simulink model "hexapod"  (R2022a)
settings: Solver=ode2  StartTime=0.0  StopTime=10.0  FixedStep=1e-4  RelTol=1e-3  AbsTol=1e-3  EnableMultiTasking=on
values from neighbouring files (symbols this model uses):
  N = 2    [gen_singleGait.m]
  s = t/T    [gait_mv_backward.m]    (also in gait_mv_forward.m; gait_mv_left.m; gait_mv_right.m; gait_rot_clockwise.m)
undefined symbols (not defined in the file or in its folder): X, Y, Z
libraries: sm_lib x90, nesl_utility x19, Contact_Forces_Lib x6, simulink x1
(part 4 of 4)

== matlab function hexapod/Leg6/MATLAB Function ==
  data: i input; ang1 output; x0 input; y0 input; z0 input; ang2 output; ang3 output; theta1 input; theta2 input; theta3 input; l1 input; l2 input; l3 input; xx1 input; yy1 input; yy2 input
function [ang1,ang2,ang3] = fcn(i,x0,y0,z0,theta1,theta2,theta3,l1,l2,l3,xx1,yy1,yy2)
p0=[x0;y0;z0];
p00=[p0;1];
j3bias=10.91;
% %
% PX=worldCo2jointCo(i,p0);
% ang=jointCo2jointAng(PX);
% ang
function TR=TROTZ(theta)
    r=theta/180*pi;
    TR=[cos(r),-sin(r),0,0;
        sin(r),cos(r),0,0;
        0,      0,    1,0;
        0,      0,    0,1];
end
function TL=TRANSL(x,y,z)
    TL=[1,0,0,x;
        0,1,0,y;
        0,0,1,z;
        0,0,0,1];
end

%%  p0->px
switch i
    case 1
        Tx_0=TROTZ(theta1)*TRANSL(-xx1,yy1,0);
    case 2
        Tx_0=TROTZ(-theta2)*TRANSL(0,-yy2,0);
    case 3
        Tx_0=TROTZ(theta3)*TRANSL(xx1,yy1,0);
    case 4
        Tx_0=TROTZ(-theta1)*TRANSL(-xx1,-yy1,0);
    case 5
        Tx_0=TROTZ(theta2)*TRANSL(0,yy2,0);
    case 6
        Tx_0=TROTZ(-theta3)*TRANSL(xx1,-yy1,0);
    otherwise
        Tx_0=zeros(4);
        disp("jijiji");
end
% Tx_0

pxx=Tx_0*p00;
px=pxx(1:3,1);
% disp(p00)
% disp(pxx)
%% px->ang
x=px(1);
y=px(2);
z=px(3);
A=sqrt(x*x+y*y)-l1;
B=-z;
if(A>0)
        assert((A*A+(z-l2)*(z-l2))>l3*l3,"not in the workspace!");
        assert((A*A+z*z)<(l2+l3)*(l2+l3),"not in the workspace!");
else
    assert((A*A+z*z)>(l3-l2)*(l3-l2),"not in the workspace!");
    assert((A*A+(z+l2)*(z+l2))<l3*l3,"not in the workspace!");
end

   

    %% 
    %   r1
    r1=atan2(y,x)*(180/pi);
        assert(r1>-60,"r1<-60, dangerous!");
        assert(r1<60,"r1>60, dangerous!");

    if((A*A+z*z)>(l2*l2+l3*l3))
%         disp("高机位捏");
            %r3
            ccos=acos((l2*l2+l3*l3-A*A-B*B)/(2*l2*l3))*(180/pi);
            if(ccos>90)
                ccos=180-ccos;
            end
            r3=180-ccos-j3bias;
                assert(r3>90-j3bias,"r3<79.09, dangerous! (might be solution of low position)");
                assert(r3<(180-j3bias),"r3>169.09, dangerous!");
            %r2
            delta=atan((l3*sin(ccos/180*pi))/(l2+(l3*cos(ccos/180*pi))));
            ttan=atan(B/A);
            r2=-90-(ttan-delta)/pi*180;
                assert(r2<0,"r2>0, dangerous!")
                assert(r2>-180,"r2<-180, dangerous!")

    else
%         disp("低机位捏");
            %   r2 
            ccos=acos((A*A+B*B+l2*l2-l3*l3)/(2*sqrt(A*A+B*B)*l2))*(180/pi);
            r2=ccos-(atan2(B,A)*(180/pi))-90;
                assert(r2>=-180,"r2<=-180, dangerous!");
                assert(r2<0,"r2>0, dangerous!");
            %   r3
            ccos2=acos((-A*A-B*B+l2*l2+l3*l3)/(2*l2*l3))*(180/pi);
                if ccos2>=90
                    ccos2=180-ccos2;
                end
            r3=ccos2-j3bias;
                assert(r3>0,"r3<0, dangerous!");
                assert(r3<(90-j3bias),"r3>79.09, dangerous!(might be solution of high position)");
                
    end

%%
ang1=r1/180*pi;
ang2=r2/180*pi;
ang3=r3/180*pi;
end

== matlab function hexapod/gait generator/前进步态/前进步态 ==
  data: x1 input; ox1 output; x2 input; z1 input; z2 input; ox2 output; ox3 output; ox4 output; ox5 output; ox6 output; oy1 output; oy2 output; oy3 output; oy4 output; oy5 output; oy6 output; oz1 output; oz2 output; oz3 output; oz4 output; oz5 output; oz6 output; xxx1 input; yyy1 input; yyy2 input; zzz1 input
function [ox1,ox2,ox3,ox4,ox5,ox6,oy1,oy2,oy3,oy4,oy5,oy6,oz1,oz2,oz3,oz4,oz5,oz6] = fcn(x1,x2,z1,z2,xxx1,yyy1,yyy2,zzz1)
% baseBias={[xxx1;-yyy1;zzz1],   [0;yyy2;zzz1],   [-xxx1;-yyy1;zzz1],...
%            [xxx1;yyy1;zzz1],    [0;-yyy2;zzz1],  [-xxx1;yyy1;zzz1]};
ox1= xxx1+x1;
ox2=      x1;
ox3=-xxx1+x1;
ox4= xxx1+x2;
ox5=      x2;
ox6=-xxx1+x2;

oy1=-yyy1;
oy2=yyy2;
oy3=-yyy1;
oy4=yyy1;
oy5=-yyy2;
oy6=yyy1;

oz1=zzz1+z1;
oz2=zzz1+z1;
oz3=zzz1+z1;
oz4=zzz1+z2;
oz5=zzz1+z2;
oz6=zzz1+z2;

== matlab function hexapod/gait generator/右移步态/步态函数 ==
  data: x1 input; ox1 output; x2 input; z1 input; z2 input; ox2 output; ox3 output; ox4 output; ox5 output; ox6 output; oy1 output; oy2 output; oy3 output; oy4 output; oy5 output; oy6 output; oz1 output; oz2 output; oz3 output; oz4 output; oz5 output; oz6 output; xxx1 input; yyy1 input; yyy2 input; zzz1 input
function [ox1,ox2,ox3,ox4,ox5,ox6,oy1,oy2,oy3,oy4,oy5,oy6,oz1,oz2,oz3,oz4,oz5,oz6] = fcn(x1,x2,z1,z2,xxx1,yyy1,yyy2,zzz1)
% baseBias={[xxx1;-yyy1;zzz1],   [0;yyy2;zzz1],   [-xxx1;-yyy1;zzz1],...
%            [xxx1;yyy1;zzz1],    [0;-yyy2;zzz1],  [-xxx1;yyy1;zzz1]};
ox1= xxx1;
ox2=0;
ox3=-xxx1;
ox4= xxx1;
ox5=0;
ox6=-xxx1;

oy1=-yyy1-x1;
oy2=yyy2-x1;
oy3=-yyy1-x1;
oy4=yyy1-x2;
oy5=-yyy2-x2;
oy6=yyy1-x2;

oz1=zzz1+z1;
oz2=zzz1+z1;
oz3=zzz1+z1;
oz4=zzz1+z2;
oz5=zzz1+z2;
oz6=zzz1+z2;

== matlab function hexapod/gait generator/后退步态/步态函数 ==
  data: x1 input; ox1 output; x2 input; z1 input; z2 input; ox2 output; ox3 output; ox4 output; ox5 output; ox6 output; oy1 output; oy2 output; oy3 output; oy4 output; oy5 output; oy6 output; oz1 output; oz2 output; oz3 output; oz4 output; oz5 output; oz6 output; xxx1 input; yyy1 input; yyy2 input; zzz1 input
function [ox1,ox2,ox3,ox4,ox5,ox6,oy1,oy2,oy3,oy4,oy5,oy6,oz1,oz2,oz3,oz4,oz5,oz6] = fcn(x1,x2,z1,z2,xxx1,yyy1,yyy2,zzz1)
% baseBias={[xxx1;-yyy1;zzz1],   [0;yyy2;zzz1],   [-xxx1;-yyy1;zzz1],...
%            [xxx1;yyy1;zzz1],    [0;-yyy2;zzz1],  [-xxx1;yyy1;zzz1]};
ox1= xxx1-x1;
ox2=     -x1;
ox3=-xxx1-x1;
ox4= xxx1-x2;
ox5=     -x2;
ox6=-xxx1-x2;

oy1=-yyy1;
oy2=yyy2;
oy3=-yyy1;
oy4=yyy1;
oy5=-yyy2;
oy6=yyy1;

oz1=zzz1+z1;
oz2=zzz1+z1;
oz3=zzz1+z1;
oz4=zzz1+z2;
oz5=zzz1+z2;
oz6=zzz1+z2;

== matlab function hexapod/gait generator/左移步态/步态函数 ==
  data: x1 input; ox1 output; x2 input; z1 input; z2 input; ox2 output; ox3 output; ox4 output; ox5 output; ox6 output; oy1 output; oy2 output; oy3 output; oy4 output; oy5 output; oy6 output; oz1 output; oz2 output; oz3 output; oz4 output; oz5 output; oz6 output; xxx1 input; yyy1 input; yyy2 input; zzz1 input
function [ox1,ox2,ox3,ox4,ox5,ox6,oy1,oy2,oy3,oy4,oy5,oy6,oz1,oz2,oz3,oz4,oz5,oz6] = fcn(x1,x2,z1,z2,xxx1,yyy1,yyy2,zzz1)
% baseBias={[xxx1;-yyy1;zzz1],   [0;yyy2;zzz1],   [-xxx1;-yyy1;zzz1],...
%            [xxx1;yyy1;zzz1],    [0;-yyy2;zzz1],  [-xxx1;yyy1;zzz1]};
ox1= xxx1;
ox2=0;
ox3=-xxx1;
ox4= xxx1;
ox5=0;
ox6=-xxx1;

oy1=-yyy1+x1;
oy2=yyy2+x1;
oy3=-yyy1+x1;
oy4=yyy1+x2;
oy5=-yyy2+x2;
oy6=yyy1+x2;

oz1=zzz1+z1;
oz2=zzz1+z1;
oz3=zzz1+z1;
oz4=zzz1+z2;
oz5=zzz1+z2;
oz6=zzz1+z2;

== matlab function hexapod/gait generator/足尖轨迹生成/x ==
  data: t input; x output; L input
function x = fcn(t,L)
%   t值域为0-1
if t<0.5
    x=L*(-16*power(t,3)+12*power(t,2)-t-1/4);
else
    x=-L*t+0.75*L;
end

== matlab function hexapod/gait generator/足尖轨迹生成/z ==
  data: t input; z output; H input
function z = fcn(t,H)
%   t值域为0-1
if t<0.5
    if t<0.25
        z=H*(-128*power(t,3)+48*power(t,2));
    else
        z=H*(-128*power((0.5-t),3)+48*power((0.5-t),2));
    end
else
    z=0;
end

== matlab function hexapod/gait generator/逆时针旋转步态/步态函数 ==
  data: x1 input; ox1 output; x2 input; z1 input; z2 input; ox2 output; ox3 output; ox4 output; ox5 output; ox6 output; oy1 output; oy2 output; oy3 output; oy4 output; oy5 output; oy6 output; oz1 output; oz2 output; oz3 output; oz4 output; oz5 output; oz6 output; xxx1 input; yyy1 input; yyy2 input; zzz1 input; L0 input; theta1 input; theta2 input; theta3 input; Ang input
function [ox1,ox2,ox3,ox4,ox5,ox6,oy1,oy2,oy3,oy4,oy5,oy6,oz1,oz2,oz3,oz4,oz5,oz6] = fcn(x1,x2,z1,z2,xxx1,yyy1,yyy2,zzz1,L0,theta1,theta2,theta3,Ang)
% baseBias={[xxx1;-yyy1;zzz1],   [0;yyy2;zzz1],   [-xxx1;-yyy1;zzz1],...
%            [xxx1;yyy1;zzz1],    [0;-yyy2;zzz1],  [-xxx1;yyy1;zzz1]};
% theta=[theta1,-theta2,theta3,-theta1,theta2,-theta3]

LL1=sqrt(xxx1*xxx1+yyy1*yyy1);
LL2=yyy2;       %sqrt(0*0+yyy2*yyy2)
L1=sqrt(2*LL1*LL1*(1-cosd(Ang)));     %4条腿的移动距离
L2=sqrt(2*LL2*LL2*(1-cosd(Ang)));     %中间2条腿的移动距离

x1_1=-x1*(L0/L1);
x2_1=-x2*(L0/L1);
z1_1=z1;
z2_1=z2;

x1_2=-x1*(L0/L2);
x2_2=-x2*(L0/L2);
z1_2=z1;
z2_2=z2;

ox1=xxx1+x1_1*sind(theta1);
oy1=-yyy1+x1_1*cosd(theta1);
oz1=zzz1+z1_1;

ox2=0+x1_2*sind(-theta2);
oy2=yyy2+x1_2*cosd(-theta2);
oz2=zzz1+z1_2;

ox3=-xxx1+x1_1*sind(theta3);
oy3=-yyy1+x1_1*cosd(theta3);
oz3=zzz1+z1_1;

ox4=xxx1+x2_1*sind(-theta1);
oy4=yyy1+x2_1*cosd(-theta1);
oz4=zzz1+z2_1;

ox5=0+x2_2*sind(theta2);
oy5=-yyy2+x2_2*cosd(theta2);
oz5=zzz1+z2_2;

ox6=-xxx1+x2_1*sind(-theta3);
oy6=yyy1+x2_1*cosd(-theta3);
oz6=zzz1+z2_1;

== matlab function hexapod/gait generator/顺时针旋转步态/步态函数 ==
  data: x1 input; ox1 output; x2 input; z1 input; z2 input; ox2 output; ox3 output; ox4 output; ox5 output; ox6 output; oy1 output; oy2 output; oy3 output; oy4 output; oy5 output; oy6 output; oz1 output; oz2 output; oz3 output; oz4 output; oz5 output; oz6 output; xxx1 input; yyy1 input; yyy2 input; zzz1 input; L0 input; theta1 input; theta2 input; theta3 input; Ang input
function [ox1,ox2,ox3,ox4,ox5,ox6,oy1,oy2,oy3,oy4,oy5,oy6,oz1,oz2,oz3,oz4,oz5,oz6] = fcn(x1,x2,z1,z2,xxx1,yyy1,yyy2,zzz1,L0,theta1,theta2,theta3,Ang)
% baseBias={[xxx1;-yyy1;zzz1],   [0;yyy2;zzz1],   [-xxx1;-yyy1;zzz1],...
%            [xxx1;yyy1;zzz1],    [0;-yyy2;zzz1],  [-xxx1;yyy1;zzz1]};
% theta=[theta1,-theta2,theta3,-theta1,theta2,-theta3]

LL1=sqrt(xxx1*xxx1+yyy1*yyy1);
LL2=yyy2;       %sqrt(0*0+yyy2*yyy2)
L1=sqrt(2*LL1*LL1*(1-cosd(Ang)));     %4条腿的移动距离
L2=sqrt(2*LL2*LL2*(1-cosd(Ang)));     %中间2条腿的移动距离

x1_1=x1*(L0/L1);
x2_1=x2*(L0/L1);
z1_1=z1;
z2_1=z2;

x1_2=x1*(L0/L2);
x2_2=x2*(L0/L2);
z1_2=z1;
z2_2=z2;

ox1=xxx1+x1_1*sind(theta1);
oy1=-yyy1+x1_1*cosd(theta1);
oz1=zzz1+z1_1;

ox2=0+x1_2*sind(-theta2);
oy2=yyy2+x1_2*cosd(-theta2);
oz2=zzz1+z1_2;

ox3=-xxx1+x1_1*sind(theta3);
oy3=-yyy1+x1_1*cosd(theta3);
oz3=zzz1+z1_1;

ox4=xxx1+x2_1*sind(-theta1);
oy4=yyy1+x2_1*cosd(-theta1);
oz4=zzz1+z2_1;

ox5=0+x2_2*sind(theta2);
oy5=-yyy2+x2_2*cosd(theta2);
oz5=zzz1+z2_2;

ox6=-xxx1+x2_1*sind(-theta3);
oy6=yyy1+x2_1*cosd(-theta3);
oz6=zzz1+z2_1;

== matlab function hexapod/Leg1/w-leg1/MATLAB Function ==
  data: i input; ang1 output; x0 input; y0 input; z0 input; ang2 output; ang3 output; theta1 input; theta2 input; theta3 input; l1 input; l2 input; l3 input; xx1 input; yy1 input; yy2 input
function [ang1,ang2,ang3] = fcn(i,x0,y0,z0,theta1,theta2,theta3,l1,l2,l3,xx1,yy1,yy2)
p0=[x0;y0;z0];
p00=[p0;1];
j3bias=10.91;
% %
% PX=worldCo2jointCo(i,p0);
% ang=jointCo2jointAng(PX);
% ang
function TR=TROTZ(theta)
    r=theta/180*pi;
    TR=[cos(r),-sin(r),0,0;
        sin(r),cos(r),0,0;
        0,      0,    1,0;
        0,      0,    0,1];
end
function TL=TRANSL(x,y,z)
    TL=[1,0,0,x;
        0,1,0,y;
        0,0,1,z;
        0,0,0,1];
end

%%  p0->px
switch i
    case 1
        Tx_0=TROTZ(theta1)*TRANSL(-xx1,yy1,0);
    case 2
        Tx_0=TROTZ(-theta2)*TRANSL(0,-yy2,0);
    case 3
        Tx_0=TROTZ(theta3)*TRANSL(xx1,yy1,0);
    case 4
        Tx_0=TROTZ(-theta1)*TRANSL(-xx1,-yy1,0);
    case 5
        Tx_0=TROTZ(theta2)*TRANSL(0,yy2,0);
    case 6
        Tx_0=TROTZ(-theta3)*TRANSL(xx1,-yy1,0);
    otherwise
        Tx_0=zeros(4);
        disp("jijiji");
end
% Tx_0

pxx=Tx_0*p00;
px=pxx(1:3,1);
% disp(p00)
% disp(pxx)
%% px->ang
x=px(1);
y=px(2);
z=px(3);
A=sqrt(x*x+y*y)-l1;
B=-z;
if(A>0)
        assert((A*A+(z-l2)*(z-l2))>l3*l3,"not in the workspace!");
        assert((A*A+z*z)<(l2+l3)*(l2+l3),"not in the workspace!");
else
    assert((A*A+z*z)>(l3-l2)*(l3-l2),"not in the workspace!");
    assert((A*A+(z+l2)*(z+l2))<l3*l3,"not in the workspace!");
end

   

    %% 
    %   r1
    r1=atan2(y,x)*(180/pi);
        assert(r1>-60,"r1<-60, dangerous!");
        assert(r1<60,"r1>60, dangerous!");

    if((A*A+z*z)>(l2*l2+l3*l3))
%         disp("高机位捏");
            %r3
            ccos=acos((l2*l2+l3*l3-A*A-B*B)/(2*l2*l3))*(180/pi);
            if(ccos>90)
                ccos=180-ccos;
            end
            r3=180-ccos-j3bias;
                assert(r3>90-j3bias,"r3<79.09, dangerous! (might be solution of low position)");
                assert(r3<(180-j3bias),"r3>169.09, dangerous!");
            %r2
            delta=atan((l3*sin(ccos/180*pi))/(l2+(l3*cos(ccos/180*pi))));
            ttan=atan(B/A);
            r2=-90-(ttan-delta)/pi*180;
                assert(r2<0,"r2>0, dangerous!")
                assert(r2>-180,"r2<-180, dangerous!")

    else
%         disp("低机位捏");
            %   r2 
            ccos=acos((A*A+B*B+l2*l2-l3*l3)/(2*sqrt(A*A+B*B)*l2))*(180/pi);
            r2=ccos-(atan2(B,A)*(180/pi))-90;
                assert(r2>=-180,"r2<=-180, dangerous!");
                assert(r2<0,"r2>0, dangerous!");
            %   r3
            ccos2=acos((-A*A-B*B+l2*l2+l3*l3)/(2*l2*l3))*(180/pi);
                if ccos2>=90
                    ccos2=180-ccos2;
                end
            r3=ccos2-j3bias;
                assert(r3>0,"r3<0, dangerous!");
                assert(r3<(90-j3bias),"r3>79.09, dangerous!(might be solution of high position)");
                
    end

%%
ang1=r1/180*pi;
ang2=r2/180*pi;
ang3=r3/180*pi;
end

== matlab function hexapod/Leg2/w-leg1/MATLAB Function ==
  data: i input; ang1 output; x0 input; y0 input; z0 input; ang2 output; ang3 output; theta1 input; theta2 input; theta3 input; l1 input; l2 input; l3 input; xx1 input; yy1 input; yy2 input
function [ang1,ang2,ang3] = fcn(i,x0,y0,z0,theta1,theta2,theta3,l1,l2,l3,xx1,yy1,yy2)
p0=[x0;y0;z0];
p00=[p0;1];
j3bias=10.91;
% %
% PX=worldCo2jointCo(i,p0);
% ang=jointCo2jointAng(PX);
% ang
function TR=TROTZ(theta)
    r=theta/180*pi;
    TR=[cos(r),-sin(r),0,0;
        sin(r),cos(r),0,0;
        0,      0,    1,0;
        0,      0,    0,1];
end
function TL=TRANSL(x,y,z)
    TL=[1,0,0,x;
        0,1,0,y;
        0,0,1,z;
        0,0,0,1];
end

%%  p0->px
switch i
    case 1
        Tx_0=TROTZ(theta1)*TRANSL(-xx1,yy1,0);
    case 2
        Tx_0=TROTZ(-theta2)*TRANSL(0,-yy2,0);
    case 3
        Tx_0=TROTZ(theta3)*TRANSL(xx1,yy1,0);
    case 4
        Tx_0=TROTZ(-theta1)*TRANSL(-xx1,-yy1,0);
    case 5
        Tx_0=TROTZ(theta2)*TRANSL(0,yy2,0);
    case 6
        Tx_0=TROTZ(-theta3)*TRANSL(xx1,-yy1,0);
    otherwise
        Tx_0=zeros(4);
        disp("jijiji");
end
% Tx_0

pxx=Tx_0*p00;
px=pxx(1:3,1);
% disp(p00)
% disp(pxx)
%% px->ang
x=px(1);
y=px(2);
z=px(3);
A=sqrt(x*x+y*y)-l1;
B=-z;
if(A>0)
        assert((A*A+(z-l2)*(z-l2))>l3*l3,"not in the workspace!");
        assert((A*A+z*z)<(l2+l3)*(l2+l3),"not in the workspace!");
else
    assert((A*A+z*z)>(l3-l2)*(l3-l2),"not in the workspace!");
    assert((A*A+(z+l2)*(z+l2))<l3*l3,"not in the workspace!");
end

   

    %% 
    %   r1
    r1=atan2(y,x)*(180/pi);
        assert(r1>-60,"r1<-60, dangerous!");
        assert(r1<60,"r1>60, dangerous!");

    if((A*A+z*z)>(l2*l2+l3*l3))
%         disp("高机位捏");
            %r3
            ccos=acos((l2*l2+l3*l3-A*A-B*B)/(2*l2*l3))*(180/pi);
            if(ccos>90)
                ccos=180-ccos;
            end
            r3=180-ccos-j3bias;
                assert(r3>90-j3bias,"r3<79.09, dangerous! (might be solution of low position)");
                assert(r3<(180-j3bias),"r3>169.09, dangerous!");
            %r2
            delta=atan((l3*sin(ccos/180*pi))/(l2+(l3*cos(ccos/180*pi))));
            ttan=atan(B/A);
            r2=-90-(ttan-delta)/pi*180;
                assert(r2<0,"r2>0, dangerous!")
                assert(r2>-180,"r2<-180, dangerous!")

    else
%         disp("低机位捏");
            %   r2 
            ccos=acos((A*A+B*B+l2*l2-l3*l3)/(2*sqrt(A*A+B*B)*l2))*(180/pi);
            r2=ccos-(atan2(B,A)*(180/pi))-90;
                assert(r2>=-180,"r2<=-180, dangerous!");
                assert(r2<0,"r2>0, dangerous!");
            %   r3
            ccos2=acos((-A*A-B*B+l2*l2+l3*l3)/(2*l2*l3))*(180/pi);
                if ccos2>=90
                    ccos2=180-ccos2;
                end
            r3=ccos2-j3bias;
                assert(r3>0,"r3<0, dangerous!");
                assert(r3<(90-j3bias),"r3>79.09, dangerous!(might be solution of high position)");
                
    end

%%
ang1=r1/180*pi;
ang2=r2/180*pi;
ang3=r3/180*pi;
end

== matlab function hexapod/Leg3/w-leg1/MATLAB Function ==
  data: i input; ang1 output; x0 input; y0 input; z0 input; ang2 output; ang3 output; theta1 input; theta2 input; theta3 input; l1 input; l2 input; l3 input; xx1 input; yy1 input; yy2 input
function [ang1,ang2,ang3] = fcn(i,x0,y0,z0,theta1,theta2,theta3,l1,l2,l3,xx1,yy1,yy2)
p0=[x0;y0;z0];
p00=[p0;1];
j3bias=10.91;
% %
% PX=worldCo2jointCo(i,p0);
% ang=jointCo2jointAng(PX);
% ang
function TR=TROTZ(theta)
    r=theta/180*pi;
    TR=[cos(r),-sin(r),0,0;
        sin(r),cos(r),0,0;
        0,      0,    1,0;
        0,      0,    0,1];
end
function TL=TRANSL(x,y,z)
    TL=[1,0,0,x;
        0,1,0,y;
        0,0,1,z;
        0,0,0,1];
end

%%  p0->px
switch i
    case 1
        Tx_0=TROTZ(theta1)*TRANSL(-xx1,yy1,0);
    case 2
        Tx_0=TROTZ(-theta2)*TRANSL(0,-yy2,0);
    case 3
        Tx_0=TROTZ(theta3)*TRANSL(xx1,yy1,0);
    case 4
        Tx_0=TROTZ(-theta1)*TRANSL(-xx1,-yy1,0);
    case 5
        Tx_0=TROTZ(theta2)*TRANSL(0,yy2,0);
    case 6
        Tx_0=TROTZ(-theta3)*TRANSL(xx1,-yy1,0);
    otherwise
        Tx_0=zeros(4);
        disp("jijiji");
end
% Tx_0

pxx=Tx_0*p00;
px=pxx(1:3,1);
% disp(p00)
% disp(pxx)
%% px->ang
x=px(1);
y=px(2);
z=px(3);
A=sqrt(x*x+y*y)-l1;
B=-z;
if(A>0)
        assert((A*A+(z-l2)*(z-l2))>l3*l3,"not in the workspace!");
        assert((A*A+z*z)<(l2+l3)*(l2+l3),"not in the workspace!");
else
    assert((A*A+z*z)>(l3-l2)*(l3-l2),"not in the workspace!");
    assert((A*A+(z+l2)*(z+l2))<l3*l3,"not in the workspace!");
end

   

    %% 
    %   r1
    r1=atan2(y,x)*(180/pi);
        assert(r1>-60,"r1<-60, dangerous!");
        assert(r1<60,"r1>60, dangerous!");

    if((A*A+z*z)>(l2*l2+l3*l3))
%         disp("高机位捏");
            %r3
            ccos=acos((l2*l2+l3*l3-A*A-B*B)/(2*l2*l3))*(180/pi);
            if(ccos>90)
                ccos=180-ccos;
            end
            r3=180-ccos-j3bias;
                assert(r3>90-j3bias,"r3<79.09, dangerous! (might be solution of low position)");
                assert(r3<(180-j3bias),"r3>169.09, dangerous!");
            %r2
            delta=atan((l3*sin(ccos/180*pi))/(l2+(l3*cos(ccos/180*pi))));
            ttan=atan(B/A);
            r2=-90-(ttan-delta)/pi*180;
                assert(r2<0,"r2>0, dangerous!")
                assert(r2>-180,"r2<-180, dangerous!")

    else
%         disp("低机位捏");
            %   r2 
            ccos=acos((A*A+B*B+l2*l2-l3*l3)/(2*sqrt(A*A+B*B)*l2))*(180/pi);
            r2=ccos-(atan2(B,A)*(180/pi))-90;
                assert(r2>=-180,"r2<=-180, dangerous!");
                assert(r2<0,"r2>0, dangerous!");
            %   r3
            ccos2=acos((-A*A-B*B+l2*l2+l3*l3)/(2*l2*l3))*(180/pi);
                if ccos2>=90
                    ccos2=180-ccos2;
                end
            r3=ccos2-j3bias;
                assert(r3>0,"r3<0, dangerous!");
                assert(r3<(90-j3bias),"r3>79.09, dangerous!(might be solution of high position)");
                
    end

%%
ang1=r1/180*pi;
ang2=r2/180*pi;
ang3=r3/180*pi;
end

== matlab function hexapod/Leg4/w-leg1/MATLAB Function ==
  data: i input; ang1 output; x0 input; y0 input; z0 input; ang2 output; ang3 output; theta1 input; theta2 input; theta3 input; l1 input; l2 input; l3 input; xx1 input; yy1 input; yy2 input
function [ang1,ang2,ang3] = fcn(i,x0,y0,z0,theta1,theta2,theta3,l1,l2,l3,xx1,yy1,yy2)
p0=[x0;y0;z0];
p00=[p0;1];
j3bias=10.91;
% %
% PX=worldCo2jointCo(i,p0);
% ang=jointCo2jointAng(PX);
% ang
function TR=TROTZ(theta)
    r=theta/180*pi;
    TR=[cos(r),-sin(r),0,0;
        sin(r),cos(r),0,0;
        0,      0,    1,0;
        0,      0,    0,1];
end
function TL=TRANSL(x,y,z)
    TL=[1,0,0,x;
        0,1,0,y;
        0,0,1,z;
        0,0,0,1];
end

%%  p0->px
switch i
    case 1
        Tx_0=TROTZ(theta1)*TRANSL(-xx1,yy1,0);
    case 2
        Tx_0=TROTZ(-theta2)*TRANSL(0,-yy2,0);
    case 3
        Tx_0=TROTZ(theta3)*TRANSL(xx1,yy1,0);
    case 4
        Tx_0=TROTZ(-theta1)*TRANSL(-xx1,-yy1,0);
    case 5
        Tx_0=TROTZ(theta2)*TRANSL(0,yy2,0);
    case 6
        Tx_0=TROTZ(-theta3)*TRANSL(xx1,-yy1,0);
    otherwise
        Tx_0=zeros(4);
        disp("jijiji");
end
% Tx_0

pxx=Tx_0*p00;
px=pxx(1:3,1);
% disp(p00)
% disp(pxx)
%% px->ang
x=px(1);
y=px(2);
z=px(3);
A=sqrt(x*x+y*y)-l1;
B=-z;
if(A>0)
        assert((A*A+(z-l2)*(z-l2))>l3*l3,"not in the workspace!");
        assert((A*A+z*z)<(l2+l3)*(l2+l3),"not in the workspace!");
else
    assert((A*A+z*z)>(l3-l2)*(l3-l2),"not in the workspace!");
    assert((A*A+(z+l2)*(z+l2))<l3*l3,"not in the workspace!");
end

   

    %% 
    %   r1
    r1=atan2(y,x)*(180/pi);
        assert(r1>-60,"r1<-60, dangerous!");
        assert(r1<60,"r1>60, dangerous!");

    if((A*A+z*z)>(l2*l2+l3*l3))
%         disp("高机位捏");
            %r3
            ccos=acos((l2*l2+l3*l3-A*A-B*B)/(2*l2*l3))*(180/pi);
            if(ccos>90)
                ccos=180-ccos;
            end
            r3=180-ccos-j3bias;
                assert(r3>90-j3bias,"r3<79.09, dangerous! (might be solution of low position)");
                assert(r3<(180-j3bias),"r3>169.09, dangerous!");
            %r2
            delta=atan((l3*sin(ccos/180*pi))/(l2+(l3*cos(ccos/180*pi))));
            ttan=atan(B/A);
            r2=-90-(ttan-delta)/pi*180;
                assert(r2<0,"r2>0, dangerous!")
                assert(r2>-180,"r2<-180, dangerous!")

    else
%         disp("低机位捏");
            %   r2 
            ccos=acos((A*A+B*B+l2*l2-l3*l3)/(2*sqrt(A*A+B*B)*l2))*(180/pi);
            r2=ccos-(atan2(B,A)*(180/pi))-90;
                assert(r2>=-180,"r2<=-180, dangerous!");
                assert(r2<0,"r2>0, dangerous!");
            %   r3
            ccos2=acos((-A*A-B*B+l2*l2+l3*l3)/(2*l2*l3))*(180/pi);
                if ccos2>=90
                    ccos2=180-ccos2;
                end
            r3=ccos2-j3bias;
                assert(r3>0,"r3<0, dangerous!");
                assert(r3<(90-j3bias),"r3>79.09, dangerous!(might be solution of high position)");
                
    end

%%
ang1=r1/180*pi;
ang2=r2/180*pi;
ang3=r3/180*pi;
end
